simulink model "PI_velocidad"  (R2015a)
settings: Solver=ode45  StartTime=0.0  StopTime=7  RelTol=1e-3
undefined symbols (not defined in the file): a, k, ki, kp
settings Model: Creator=HP  LastModifiedBy=HP

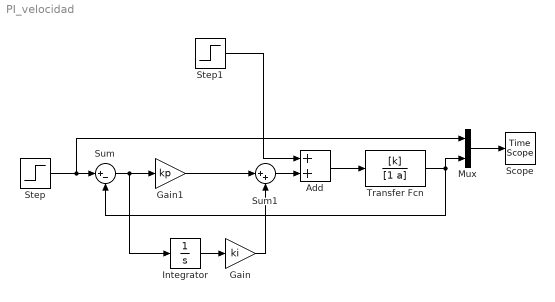
== system PI_velocidad ==
  Add : Sum
  Gain : Gain  Gain=ki
  Gain1 : Gain  Gain=kp
  Integrator : Integrator
  Mux : Mux  Inputs=2
  Scope : TimeScope
  Step : Step  Time=0  SampleTime=0
  Step1 : Step  Time=3  After=-.25  SampleTime=0
  Sum : Sum  Inputs=|+-
  Sum1 : Sum  Inputs=|++
  Transfer Fcn : TransferFcn  Numerator=[k]  Denominator=[1 a]
  wires:
  Step/1 -> Mux/1, Sum/1
  Sum/1 -> Integrator/1, Gain1/1
  Gain1/1 -> Sum1/1
  Integrator/1 -> Gain/1
  Gain/1 -> Sum1/2
  Add/1 -> Transfer Fcn/1
  Sum1/1 -> Add/2
  Transfer Fcn/1 -> Mux/2, Sum/2
  Mux/1 -> Scope/1
  Step1/1 -> Add/1
